simulink model "pendulumgui"  (R2016a)
settings: Solver=ode4  StartTime=0.0  StopTime=20  FixedStep=0.001  RelTol=1e-3
values from neighbouring files (symbols this model uses):
  c1 = str2double(sys_parameters{6})    [DIP_gui.m]    (also in paramters.m = 0.0001)
  c2 = str2double(sys_parameters{12})    [DIP_gui.m]    (also in paramters.m = 0.002)
  g = -9.8    [BP_linear.m]    (also in DIP_gui.m = str2double(sys_parameters{13}); paramters.m = 9.8)
  I1 = str2double(sys_parameters{5})    [DIP_gui.m]    (also in paramters.m = 0.0089)
  I2 = str2double(sys_parameters{11})    [DIP_gui.m]    (also in paramters.m = 0.0018)
  Jn1 = str2double(sys_parameters{4})    [DIP_gui.m]    (also in paramters.m = 2.8e-05)
  Jn2 = str2double(sys_parameters{10})    [DIP_gui.m]    (also in paramters.m = 2e-06)
  L = str2double(sys_parameters{14})    [DIP_gui.m]    (also in paramters.m = 0.38)
  l1 = str2double(sys_parameters{3})    [DIP_gui.m]    (also in paramters.m = 0.19)
  l2 = str2double(sys_parameters{9})    [DIP_gui.m]    (also in paramters.m = 0.115)
  m1 = str2double(sys_parameters{1})    [DIP_gui.m]    (also in paramters.m = 0.18)
  m2 = str2double(sys_parameters{7})    [DIP_gui.m]    (also in paramters.m = 0.1)
  n1 = str2double(sys_parameters{2})    [DIP_gui.m]    (also in paramters.m = 0.078)
  n2 = str2double(sys_parameters{8})    [DIP_gui.m]    (also in paramters.m = 0.05)
  T = 0.01    [paramters.m]
undefined symbols (not defined in the file or in its folder): a1, a2, m0
libraries: vrlib x6, simulink x1
settings Model: Creator=akhan  LastModifiedBy=akhan
settings SolverCC: SolverResetMethod=Robust
settings DataIOCC: LimitDataPoints=on  SaveFormat=Array
settings OptimizationCC: SimCompilerOptimization=on
settings DebuggingCC: SolverPrmCheckMsg=warning  MultiTaskRateTransMsg=warning
settings HardwareCC: ProdBitPerPointer=32  ProdLargestAtomicFloat=None  ProdIntDivRoundTo=Undefined  ProdEndianess=Unspecified  ProdWordSize=32  ProdHWDeviceType=32-bit Generic
settings ModelReferenceCC: PropagateSignalLabelsOutOfModel=off
settings ConfigComp: CovModelRefEnable=Off  CovSFcnEnable=off

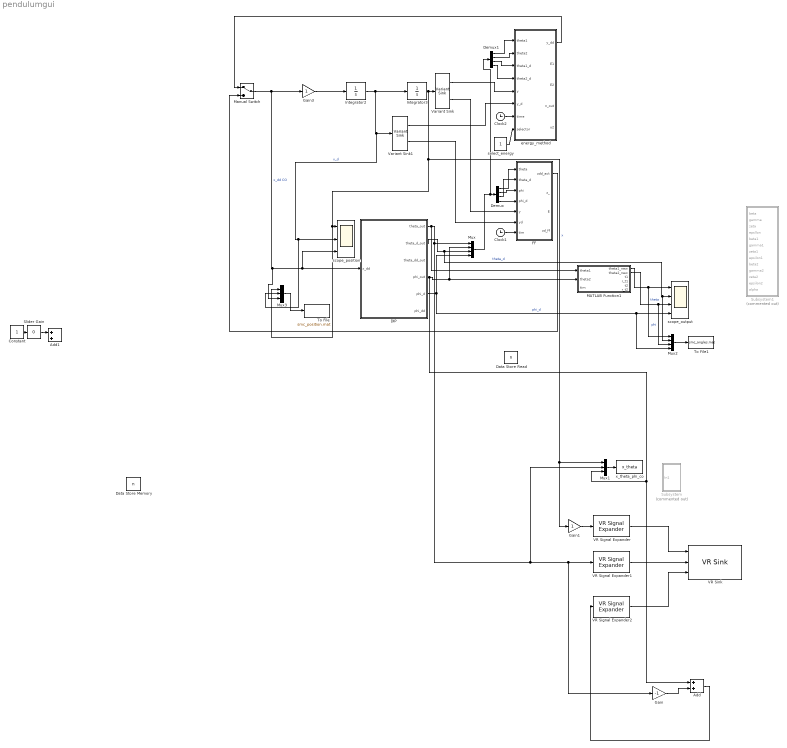
== system pendulumgui ==
  Add : Sum
  Add1 : Sum
  Clock1 : Clock
  Clock2 : Clock
  Constant : Constant
  DIP : Subsystem
  Data Store Memory : DataStoreMemory  DataStoreName=n  InitialValue=1  ShowAdditionalParam=off  OutDataTypeStr=double
  Data Store Read : DataStoreRead  DataStoreName=n  DataStoreElements=n
  Demux : Demux
  Demux1 : Demux
  FF : Subsystem
  Gain : Gain  Gain=-1
  Gain1 : Gain
  Gain3 : Gain
  Integrator2 : Integrator
  Integrator3 : Integrator  LimitOutput=on  UpperSaturationLimit=8  LowerSaturationLimit=-8
  MATLAB Function1 : MATLAB Function  TreatAsAtomicUnit=on
  Manual Switch : ManualSwitch
  Mux : Mux
  Mux1 : Mux  Inputs=3
  Mux2 : Mux
  Mux3 : Mux  Inputs=3
  Slider Gain : simulink/Math Operations/Slider Gain  low=-50  gain=0  high=50
  Subsystem : Subsystem  Commented=on
  Subsystem1 : Subsystem  Commented=on  mask{m0=0.8, m1=0.18, m2=0.10, l1=0.19, l2=0.115, a1=0.01, c1=0.2, a2=0.01, c2=0.2, g=9.8}
  To File : ToFile  Filename=smc_position.mat  SaveFormat=Timeseries
  To File1 : ToFile  Filename=smc_angles.mat  SaveFormat=Timeseries
  VR Signal Expander : vrlib/VR Signal Expander  outwidth=3  outidx=[1]
  VR Signal Expander1 : vrlib/VR Signal Expander  outwidth=4  outidx=[4]
  VR Signal Expander2 : vrlib/VR Signal Expander  outwidth=4  outidx=[4]
  VR Sink : vrlib/VR Sink  InstantiateOnLoad=on  SampleTime=0.05  ViewEnable=on  RemoteChange=off  RemoteView=off  FieldsWritten=slider_wpendulum.translation.3.1.1.double#first_arm.rotation.4.1.1.double#second_arm.rotation.4.1.1.double  WorldFileName=Double_Inverted_Pendullum_updated3.wrl  AutoView=off  VideoDimensions=[]  AllowVariableSize=off
  Variant Sink : VariantSink  ShowConditionOnBlock=on
  Variant Sink1 : VariantSink
  energy_method : MATLAB Function  TreatAsAtomicUnit=on
  scope_output : Scope  NumInputPorts=4
  scope_position : Scope  NumInputPorts=3
  select_energy : Constant
  x_theta_phi_co : ToWorkspace  VariableName=x_theta  SaveFormat=Timeseries  SampleTime=-1
  wires:
  Add/1 -> VR Signal Expander2/1
  Gain/1 -> Add/2
  DIP/4(phi_out) -> Mux1/3, Add/1, Mux/2, MATLAB Function1/2(theta2)
  Gain3/1 -> Integrator2/1
  DIP/5(phi_d) -> Mux/4, Mux2/4, scope_output/4  "phi_d"
  Constant/1 -> Slider Gain/1
  Slider Gain/1 -> Add1/1
  MATLAB Function1/2(theta2_new) -> Mux2/3, scope_output/3  "phi"
  select_energy/1 -> energy_method/8(selector)
  DIP/2(theta_d_out) -> Mux2/2, scope_output/2, Mux/3  "theta_d"
  Mux/1 -> Demux/1, Demux1/1
  Clock1/1 -> FF/7(tim)
  Clock2/1 -> energy_method/7(time)
  Demux1/1 -> energy_method/1(theta1)
  Demux1/2 -> energy_method/2(theta2)
  Demux1/3 -> energy_method/3(theta1_d)
  Demux1/4 -> energy_method/4(theta2_d)
  Variant Sink/1 -> energy_method/5(y)
  Variant Sink1/1 -> energy_method/6(y_d)
  Integrator2/1 -> Mux3/2, scope_position/2, Variant Sink1/1, Integrator3/1  "x_d"
  Manual Switch/1 -> Mux3/3, scope_position/3, DIP/1(x_dd), Gain3/1  "x_dd CO"
  energy_method/1(y_dd) -> Manual Switch/1
  DIP/1(theta_out) -> Mux/1, Mux1/2, Gain/1, VR Signal Expander1/1, MATLAB Function1/1(theta1)
  Integrator3/1 -> Mux3/1, scope_position/1, Mux1/1, Gain1/1, Variant Sink/1  "x"
  Variant Sink1/2 -> FF/6(yd)
  Demux/1 -> FF/1(theta)
  Demux/3 -> FF/2(theta_d)
  Demux/2 -> FF/3(phi)
  Demux/4 -> FF/4(phi_d)
  Variant Sink/2 -> FF/5(y)
  FF/1(zdd_act) -> Manual Switch/2
  Mux1/1 -> x_theta_phi_co/1
  VR Signal Expander/1 -> VR Sink/1
  VR Signal Expander1/1 -> VR Sink/2
  VR Signal Expander2/1 -> VR Sink/3
  Gain1/1 -> VR Signal Expander/1
  MATLAB Function1/1(theta1_new) -> Mux2/1, scope_output/1  "theta"
  Mux2/1 -> To File1/1
  Mux3/1 -> To File/1

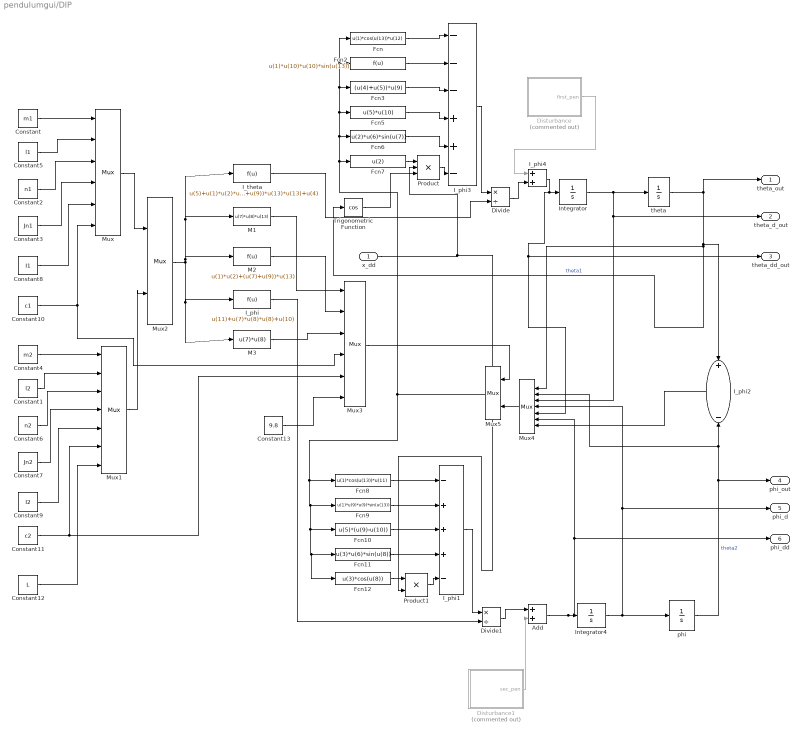
== system pendulumgui/DIP ==
  x_dd : Inport
  Add : Sum
  Constant : Constant  Value=m1
  Constant1 : Constant  Value=l2
  Constant10 : Constant  Value=c1
  Constant11 : Constant  Value=c2
  Constant12 : Constant  Value=L
  Constant13 : Constant  Value=9.8
  Constant2 : Constant  Value=n1
  Constant3 : Constant  Value=Jn1
  Constant4 : Constant  Value=m2
  Constant5 : Constant  Value=l1
  Constant6 : Constant  Value=n2
  Constant7 : Constant  Value=Jn2
  Constant8 : Constant  Value=I1
  Constant9 : Constant  Value=I2
  Disturbance : Subsystem  Commented=on
  Disturbance1 : Subsystem  Commented=on
  Divide : Product  Inputs=*/
  Divide1 : Product  Inputs=*/
  Fcn : Fcn  Expr=u(1)*cos(u(13))*u(12)
  Fcn10 : Fcn  Expr=u(5)*(u(9)-u(10))
  Fcn11 : Fcn  Expr=u(3)*u(6)*sin(u(8))
  Fcn12 : Fcn  Expr=u(3)*cos(u(8))
  Fcn2 : Fcn  Expr=u(1)*u(10)*u(10)*sin(u(13))
  Fcn3 : Fcn  Expr=(u(4)+u(5))*u(9)
  Fcn5 : Fcn  Expr=u(5)*u(10)
  Fcn6 : Fcn  Expr=u(2)*u(6)*sin(u(7))
  Fcn7 : Fcn  Expr=u(2)
  Fcn8 : Fcn  Expr=u(1)*cos(u(13))*u(11)
  Fcn9 : Fcn  Expr=u(1)*u(9)*u(9)*sin(u(13))
  I_phi : Fcn  Expr=u(11)+u(7)*u(8)*u(8)+u(10)
  I_phi1 : Sum  Inputs=-+++-
  I_phi2 : Sum  Inputs=+|-
  I_phi3 : Sum  Inputs=---++-
  I_phi4 : Sum
  I_theta : Fcn  Expr=u(5)+u(1)*u(2)*u(2)+(u(7)+u(9))*u(13)*u(13)+u(4)
  Integrator : Integrator
  Integrator4 : Integrator
  M1 : Fcn  Expr=u(7)*u(8)*u(13)
  M2 : Fcn  Expr=u(1)*u(2)+(u(7)+u(9))*u(13)
  M3 : Fcn  Expr=u(7)*u(8)
  Mux : Mux  Inputs=6
  Mux1 : Mux  Inputs=7
  Mux2 : Mux  Inputs=2
  Mux3 : Mux  Inputs=6
  Mux4 : Mux  Inputs=7
  Mux5 : Mux  Inputs=2
  Product : Product  Inputs=3
  Product1 : Product
  Trigonometric Function : Trigonometry  Operator=cos
  phi : Integrator  InitialCondition=-pi  WrapState=on
  theta : Integrator  InitialCondition=-pi+(pi/100)  WrapState=on
  theta_out : Outport
  theta_d_out : Outport  Port=2
  theta_dd_out : Outport  Port=3
  phi_out : Outport  Port=4
  phi_d : Outport  Port=5
  phi_dd : Outport  Port=6
  wires:
  Integrator4/1 -> Mux4/4, phi_d/1, phi/1
  Integrator/1 -> Mux4/3, theta_d_out/1, theta/1
  theta/1 -> Trigonometric Function/1, Mux4/1, I_phi2/1, theta_out/1  "theta1"
  phi/1 -> Mux4/2, I_phi2/2, phi_out/1  "theta2"
  Constant/1 -> Mux/1
  Constant5/1 -> Mux/2
  Constant2/1 -> Mux/3
  Constant3/1 -> Mux/4
  Constant8/1 -> Mux/5
  Constant10/1 -> Mux/6, Mux3/4
  Constant4/1 -> Mux1/1
  Constant1/1 -> Mux1/2
  Constant6/1 -> Mux1/3
  Constant7/1 -> Mux1/4
  Constant9/1 -> Mux1/5
  Constant11/1 -> Mux3/5, Mux1/6
  Mux/1 -> Mux2/1
  Mux1/1 -> Mux2/2
  Mux2/1 -> M3/1, I_phi/1, M2/1, I_theta/1, M1/1
  Constant12/1 -> Mux1/7
  M1/1 -> Mux3/1
  M2/1 -> Mux3/2
  M3/1 -> Mux3/3
  Constant13/1 -> Mux3/6
  I_phi3/1 -> Divide/1
  I_theta/1 -> Divide/2
  I_phi/1 -> Divide1/2
  Mux4/1 -> Mux5/2
  Mux3/1 -> Mux5/1
  I_phi1/1 -> Divide1/1
  Fcn/1 -> I_phi3/1
  Fcn2/1 -> I_phi3/2
  Fcn3/1 -> I_phi3/3
  Fcn5/1 -> I_phi3/4
  Fcn6/1 -> I_phi3/5
  Mux5/1 -> Fcn10/1, Fcn11/1, Fcn12/1, Fcn9/1, Fcn8/1, Fcn/1, Fcn2/1, Fcn3/1, Fcn5/1, Fcn6/1, Fcn7/1
  Fcn8/1 -> I_phi1/1
  Fcn9/1 -> I_phi1/2
  Fcn10/1 -> I_phi1/3
  Fcn11/1 -> I_phi1/4
  I_phi2/1 -> Mux4/7
  Product/1 -> I_phi3/6
  Fcn12/1 -> Product1/1
  Product1/1 -> I_phi1/5
  x_dd/1 -> Product1/2, Product/2
  Trigonometric Function/1 -> Product/3
  Fcn7/1 -> Product/1
  I_phi4/1 -> Mux4/5, theta_dd_out/1, Integrator/1
  Add/1 -> phi_dd/1, Mux4/6, Integrator4/1
  Divide1/1 -> Add/1
  Divide/1 -> I_phi4/2
  Disturbance/1(first_pen) -> I_phi4/1
  Disturbance1/1(sec_pen) -> Add/2

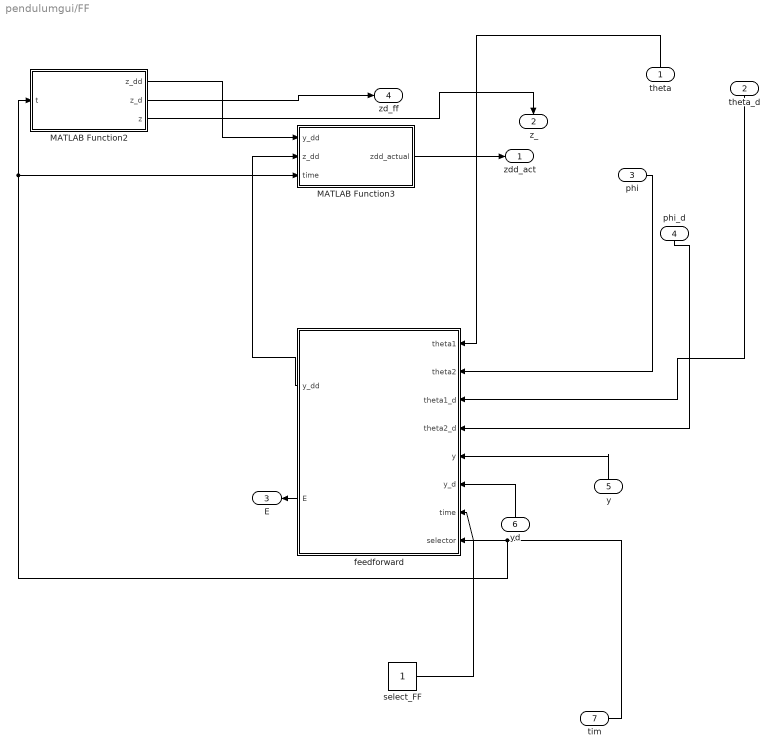
== system pendulumgui/FF ==
  theta : Inport
  theta_d : Inport  Port=2
  phi : Inport  Port=3
  phi_d : Inport  Port=4
  y : Inport  Port=5
  yd : Inport  Port=6
  tim : Inport  Port=7
  MATLAB Function2 : MATLAB Function  TreatAsAtomicUnit=on
  MATLAB Function3 : MATLAB Function  TreatAsAtomicUnit=on
  feedforward : MATLAB Function  TreatAsAtomicUnit=on
  select_FF : Constant
  zdd_act : Outport
  z_ : Outport  Port=2
  E : Outport  Port=3
  zd_ff : Outport  Port=4
  wires:
  feedforward/2(E) -> E/1
  y/1 -> feedforward/5(y)
  phi_d/1 -> feedforward/4(theta2_d)
  theta_d/1 -> feedforward/3(theta1_d)
  phi/1 -> feedforward/2(theta2)
  yd/1 -> feedforward/6(y_d)
  theta/1 -> feedforward/1(theta1)
  tim/1 -> MATLAB Function3/3(time), MATLAB Function2/1(t), feedforward/7(time)
  MATLAB Function3/1(zdd_actual) -> zdd_act/1
  MATLAB Function2/2(z_d) -> zd_ff/1
  MATLAB Function2/1(z_dd) -> MATLAB Function3/1(y_dd)
  MATLAB Function2/3(z) -> z_/1
  feedforward/1(y_dd) -> MATLAB Function3/2(z_dd)
  select_FF/1 -> feedforward/8(selector)

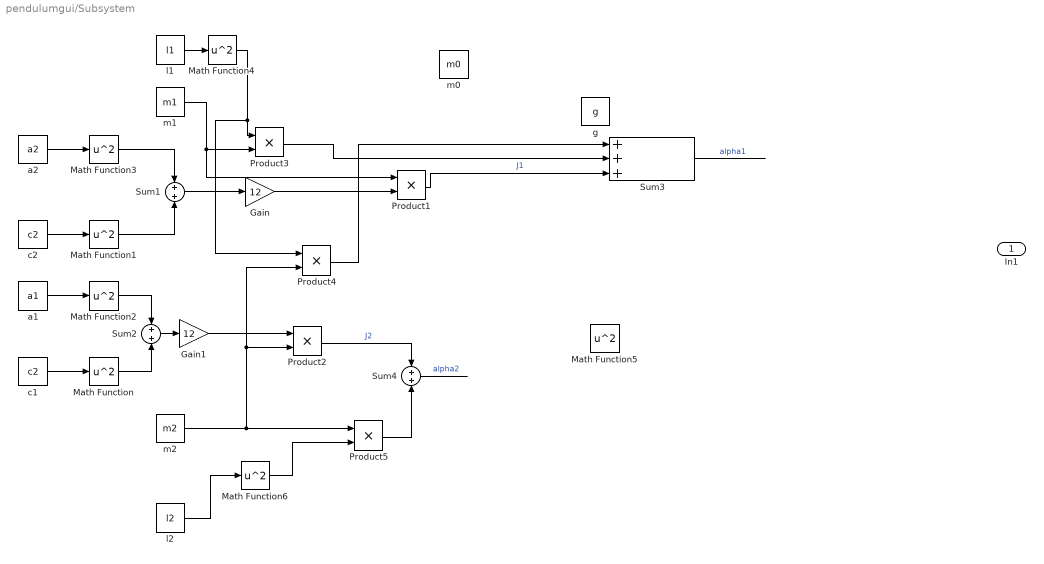
== system pendulumgui/Subsystem ==
  In1 : Inport
  Gain : Gain  Gain=12
  Gain1 : Gain  Gain=12
  Math Function{,1..6} (7 alike) : Math  Operator=square  SaturateOnIntegerOverflow=on
  Product{1..5} (5 alike) : Product
  Sum1 : Sum  Inputs=+|+
  Sum2 : Sum  Inputs=+|+
  Sum3 : Sum  Inputs=+++
  Sum4 : Sum  Inputs=+|+
  a1 : Constant  Value=a1
  a2 : Constant  Value=a2
  c1 : Constant  Value=c2
  c2 : Constant  Value=c2
  g : Constant  Value=g
  l1 : Constant  Value=l1
  l2 : Constant  Value=l2
  m0 : Constant  Value=m0
  m1 : Constant  Value=m1
  m2 : Constant  Value=m2
  wires:
  a2/1 -> Math Function3/1
  a1/1 -> Math Function2/1
  c2/1 -> Math Function1/1
  Math Function3/1 -> Sum1/1
  Math Function/1 -> Sum2/2
  Math Function1/1 -> Sum1/2
  Math Function2/1 -> Sum2/1
  m2/1 -> Product4/2, Product2/2, Product5/1
  m1/1 -> Product1/1, Product3/2
  c1/1 -> Math Function/1
  Product1/1 -> Sum3/3  "J1"
  Product3/1 -> Sum3/2
  l1/1 -> Math Function4/1
  Math Function4/1 -> Product4/1, Product3/1
  Product4/1 -> Sum3/1
  Sum3/1 -> ?  "alpha1"
  l2/1 -> Math Function6/1
  Sum1/1 -> Gain/1
  Gain/1 -> Product1/2
  Sum2/1 -> Gain1/1
  Gain1/1 -> Product2/1
  Math Function6/1 -> Product5/2
  Product2/1 -> Sum4/1  "J2"
  Product5/1 -> Sum4/2
  Sum4/1 -> ?  "alpha2"

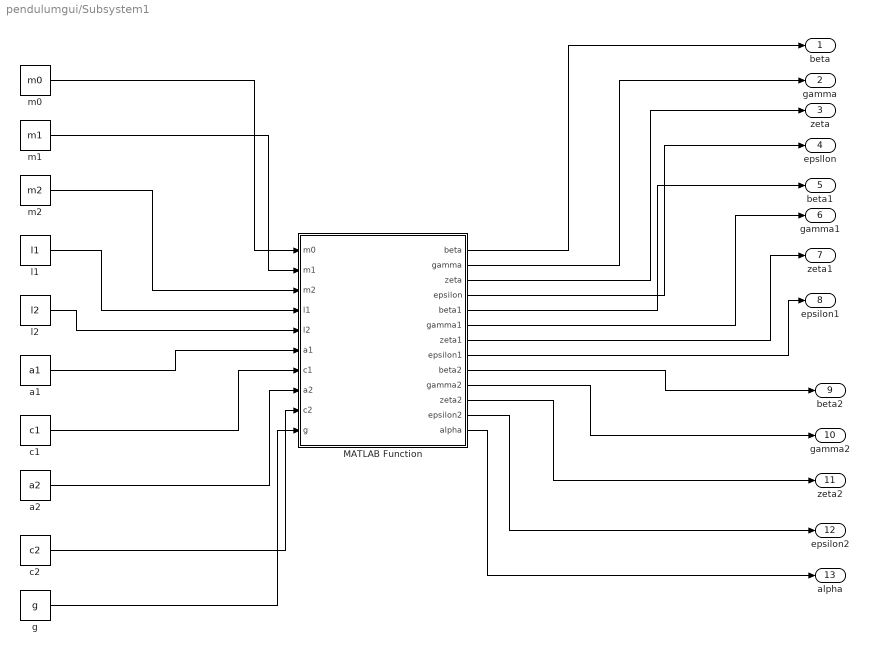
== system pendulumgui/Subsystem1 ==
  MATLAB Function : MATLAB Function  TreatAsAtomicUnit=on
  a1 : Constant  Value=a1
  a2 : Constant  Value=a2
  c1 : Constant  Value=c1
  c2 : Constant  Value=c2
  g : Constant  Value=g
  "l1 " : Constant  Value=l1
  l2 : Constant  Value=l2
  m0 : Constant  Value=m0
  m1 : Constant  Value=m1
  m2 : Constant  Value=m2
  beta : Outport
  gamma : Outport  Port=2
  zeta : Outport  Port=3
  epsllon : Outport  Port=4
  beta1 : Outport  Port=5
  gamma1 : Outport  Port=6
  zeta1 : Outport  Port=7
  epsilon1 : Outport  Port=8
  beta2 : Outport  Port=9
  gamma2 : Outport  Port=10
  zeta2 : Outport  Port=11
  epsilon2 : Outport  Port=12
  alpha : Outport  Port=13
  wires:
  m1/1 -> MATLAB Function/2(m1)
  m0/1 -> MATLAB Function/1(m0)
  "l1 "/1 -> MATLAB Function/4(l1)
  c2/1 -> MATLAB Function/9(c2)
  MATLAB Function/1(beta) -> beta/1
  MATLAB Function/10(gamma2) -> gamma2/1
  MATLAB Function/11(zeta2) -> zeta2/1
  MATLAB Function/5(beta1) -> beta1/1
  MATLAB Function/12(epsilon2) -> epsilon2/1
  MATLAB Function/9(beta2) -> beta2/1
  MATLAB Function/2(gamma) -> gamma/1
  MATLAB Function/7(zeta1) -> zeta1/1
  MATLAB Function/6(gamma1) -> gamma1/1
  MATLAB Function/3(zeta) -> zeta/1
  MATLAB Function/4(epsilon) -> epsllon/1
  MATLAB Function/8(epsilon1) -> epsilon1/1
  m2/1 -> MATLAB Function/3(m2)
  l2/1 -> MATLAB Function/5(l2)
  a1/1 -> MATLAB Function/6(a1)
  c1/1 -> MATLAB Function/7(c1)
  a2/1 -> MATLAB Function/8(a2)
  g/1 -> MATLAB Function/10(g)
  MATLAB Function/13(alpha) -> alpha/1

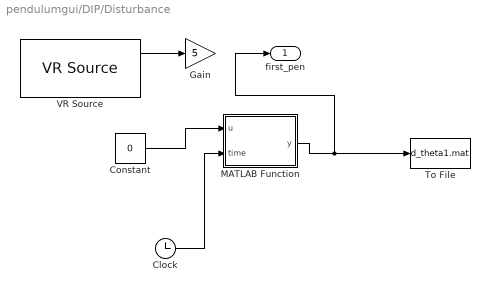
== system pendulumgui/DIP/Disturbance ==
  Clock : Clock
  Constant : Constant  Value=0
  Gain : Gain  Gain=5
  MATLAB Function : MATLAB Function  TreatAsAtomicUnit=on
  To File : ToFile  Filename=d_theta1.mat  SaveFormat=Timeseries
  VR Source : vrlib/VR Source  InstantiateOnLoad=on  SampleTime=T  ViewEnable=on  RemoteChange=off  RemoteView=off  FieldsRead=first_arm_touch.isActive#second_arm_touch.isActive  WorldFileName=Double_Inverted_Pendullum_updated3.wrl  AutoView=off  VideoDimensions=[]  AllowVariableSize=off
  first_pen : Outport
  wires:
  VR Source/1 -> Gain/1
  MATLAB Function/1(y) -> first_pen/1, To File/1
  Constant/1 -> MATLAB Function/1(u)
  Clock/1 -> MATLAB Function/2(time)

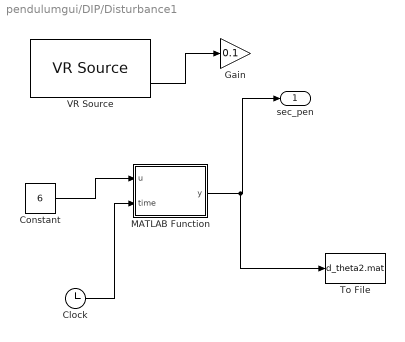
== system pendulumgui/DIP/Disturbance1 ==
  Clock : Clock
  Constant : Constant  Value=6
  Gain : Gain  Gain=0.1  OutDataTypeStr=double
  MATLAB Function : MATLAB Function  TreatAsAtomicUnit=on
  To File : ToFile  Filename=d_theta2.mat  SaveFormat=Timeseries
  VR Source : vrlib/VR Source  InstantiateOnLoad=on  SampleTime=T  ViewEnable=on  RemoteChange=off  RemoteView=off  FieldsRead=first_arm_touch.isActive.1.1.1.logical#second_arm_touch.isActive.1.1.1.logical  WorldFileName=Double_Inverted_Pendullum_updated3.wrl  AutoView=off  VideoDimensions=[]  AllowVariableSize=off
  sec_pen : Outport
  wires:
  VR Source/2 -> Gain/1
  Constant/1 -> MATLAB Function/1(u)
  Clock/1 -> MATLAB Function/2(time)
  MATLAB Function/1(y) -> To File/1, sec_pen/1

== matlab function pendulumgui/DIP/Disturbance/MATLAB Function ==
  data: u input; y output; time input
function y = fcn(u,time)
%#codegen
if time>5&&time<6
y = u;
else
    y=0;
end

== matlab function pendulumgui/Subsystem1/MATLAB Function ==
  data: m0 input; beta output; m1 input; m2 input; l1 input; l2 input; a1 input; c1 input; a2 input; c2 input; g input; gamma output; zeta output; epsilon output; beta1 output; gamma1 output; zeta1 output; epsilon1 output; beta2 output; gamma2 output; zeta2 output; epsilon2 output; alpha output
function [beta,gamma,zeta,epsilon,beta1,gamma1,zeta1,epsilon1,beta2,gamma2,zeta2,epsilon2,alpha] = fcn(m0,m1,m2,l1,l2,a1,c1,a2,c2,g)
%#codegen
J1=m1*((a1*a1)+(c1*c1))/12;
J2=m2*((a2*a2)+(c2*c2))/12;
J1=0.0089;
J2=0.0018;
alpha1 = (m1*l1*l1)+(m2*l1*l1)+J1;
alpha2 = (m2*l2*l2)+J2;

beta1 = (m1*l1)+(m2*l1);
beta2 = m2*l2;

gamma1 = m2*l1*l2;
gamma2 = gamma1;

zeta1 = gamma1;
zeta2 = gamma1;

epsilon1 = ((m1*l1)+(m2*l1))*g;
epsilon2 = beta2;

alpha = m0+m1+m2;
beta = beta1;
gamma = epsilon2;
zeta = beta;
epsilon = gamma;

beta1 = beta1/alpha1;
gamma1 = gamma1/alpha1;
zeta1 = zeta1/alpha1;
epsilon1 = epsilon1/alpha1;

beta2 = beta2/alpha2;
gamma2 = gamma2/alpha2;
zeta2 = zeta2/alpha2;
epsilon2 = epsilon2/alpha2;

beta = beta/alpha;
gamma = gamma/alpha;
zeta = zeta/alpha;
epsilon = epsilon/alpha;

== matlab function pendulumgui/MATLAB Function1 ==
  data: theta1 input; theta1_new output; theta2 input; theta2_new output; t1 output; r_t1 output; t2 output; r_t2 output; tim input
function [theta1_new,theta2_new,t1,r_t1,t2,r_t2] = fcn(theta1,theta2,tim)
%#codegen

theta1_new = cos(theta1);
theta1_new = acosd(theta1_new);
theta2_new = cos(theta2);
theta2_new = acosd(theta2_new);


% if theta1>2*pi||theta1<(-2*pi)
%     t1 = mod(theta1,2*pi);
%     r_t1 = 1;
% else r_t1 =0;
%     t1 = theta1;
% end
% 
% if theta2>2*pi||theta2<(-2*pi)
%     t2 = mod(theta2,2*pi);
%     r_t2 = 1;
% else r_t2 =0;
%     t2 = theta2;
% end

if tim==0
    r_t1 = 1;
    r_t2 = 1;
   t1 = 0;
   t2 = 0;
else
    r_t1=0;
    r_t2=0;
    t1=0;
    t2=0;
end

== matlab function pendulumgui/DIP/Disturbance1/MATLAB Function ==
  data: u input; y output; time input
function y = fcn(u,time)
%#codegen
if time>5&&time<7
y = u;
else
    y=0;
end

== matlab function pendulumgui/FF/feedforward ==
  data: theta1 input; theta2 input; theta1_d input; theta2_d input; y input; y_d input; y_dd output; time input; E output; selector input
function [y_dd,E] =fcn(theta1,theta2,theta1_d,theta2_d,y,y_d,time,selector)
%#codegen

m1 = 0.18;
n1 = 0.078;
l1 = 0.19;
Jn1 = 2.8e-5;
I1 = 0.0089;
c1 = 0.0001;
m2 = 0.1;
n2 = 0.05;
l2 = 0.115;
Jn2 = 2e-6;
I2 = 0.0018;
c2 = 0.002;
g = 9.8;
L = 0.38;
alpha_theta = 1;
alpha_phi = 2;
alpha_theta_d = 1.2;
alpha_phi_d = 20;

E = alpha_theta*abs(theta1)+alpha_phi*abs(theta2);
E = alpha_theta_d*abs(theta1_d)+alpha_phi_d*abs(theta2_d);
E1 = 1/2*I1*theta1_d^2;
E1 = E1 + m1*g*l1*(cos(theta1)-1);

E2 = 1/2*I2*theta2_d^2;
E2 = E2 + m2*g*l2*(cos(theta2)-1);

I_theta = I1 +m1*(l1^2)+m2*(L^2)+n2*(L^2)+Jn1;
M1 = m2*l2*L;
M2 = m1*l1+m2*L+n2*L;
I_phi = I2+m2*(l2*l2)+Jn2;
M3=m2*l2;

%Calculating energy

t_exit=15;
ua1 = 14;
%X_dd in first phase



if time>1.6
    n_out = 3;
x3 = [theta1;theta1_d;theta2;theta2_d;y;y_d];

a21 = -M2*I_phi*g;
a_den =(I_phi*I_theta-(M1^2));
a21 = a21/a_den;

a22 = -(M1*c2+I_phi*(c1+c2));
a22 = a22/a_den;

a23 = M1*M3*g/a_den;

a24 = I_phi*c1 + M1*c2;
a24 = a24/a_den;

a41 = M1*M2*g/a_den;

a42 = I_theta*c2 + M1*(c1+c2);
a42 = a42/a_den;


a43 = -(M3*I_theta)*g/a_den;

a44 = -(I_theta*c2+M1*c1);
a44 = a44/a_den;

b2 = M1*M3-M2*I_phi;
b2 = b2/a_den;

b4 = M1*M2-M3*I_theta;
b4 = b4/a_den;

A3 = [0 1 0 0 0 0
     a21 a22 a23 a24 0 0
     0 0 0 1 0 0
     a41 a42 a43 a44 0 0
     0 0 0 0 0 1
     0 0 0 0 0 0];
 B3 = [0;b2;0;b4;0;1];
    A3 =[         0    1.0000         0         0         0         0
   28.8552   -0.1581   -5.0889    0.1549         0         0
         0         0         0    1.0000         0         0
  -40.3575    0.8612   43.1873   -0.8567         0         0
         0         0         0         0         0         1
         0         0         0         0         0         0];
 
 ep3 = 1;
 K3 = 10;
 R3=3;
 
% P3 = care(A3+ep3*eye(6),B3,eye(6));


P3 = 1.0e+03 *[3.3164    0.0753   -5.1074   -0.7356   -0.1996   -0.2951
                0.0753    0.0099   -0.0443   -0.0057    0.0097    0.0097
               -5.1074   -0.0443    8.5062    1.2307    0.4325    0.5997
               -0.7356   -0.0057    1.2307    0.1782    0.0634    0.0877
               -0.1996    0.0097    0.4325    0.0634    0.0506    0.0518
               -0.2951    0.0097    0.5997    0.0877    0.0518    0.0641];


S3 = (B3')*P3;


sigma_3 = S3*x3;

u3_1 = -inv(S3*B3);
u3_2 = S3*A3*x3;
u3_3 = R3*sign(sigma_3);
u3_4 = K3*sigma_3;
u3 = u3_1*(u3_2+u3_3+u3_4);
% gain = -[ -81.4700   -7.0211   76.8723   10.3521    0.1513    0.4473];
gain = -[ -360.2187  -19.7350  431.6744   65.4821    3.1623    7.3102];
%0 IS SMC and anything else is LQR
if selector==0
    y_dd = u3;
else
    y_dd = gain*x3; 
end

u2 = 0;
else
    y_dd = 0;
    n_out = 3;
    u2= 0;
    
end

== matlab function pendulumgui/FF/MATLAB Function2 ==
  data: t input; z_dd output; z_d output; z output
function [z_dd,z_d,z]  = fcn(t)
%#codegen



% p =[   -0.2007
%     0.1709
%     0.3038
%     0.1094];
% T = 1.8;


p=[  0.0859
    0.1996
   -0.0939
   -0.1516];
T=2.2;
if t==2.5
    j=5;
end
a0 = -p(1)-p(3);
a1 = -p(2)-p(4);

z = a0+a1*cos(pi*t/T);
z_d = (-a1*pi/T)*sin(pi*t/T);
z_dd = (-a1*pi*pi/T^2)*cos(pi*t/T);

for i=2:5
    z = z + p(i-1)*cos(i*pi*t/T);
    z_d = z_d -(p(i-1)*i*pi/T)*sin(i*pi*t/T);
    z_dd = z_dd-(p(i-1)*i*i*pi*pi/T^2)*cos(i*pi*t/T);
end

end

== matlab function pendulumgui/FF/MATLAB Function3 ==
  data: y_dd input; zdd_actual output; z_dd input; time input
function zdd_actual  = fcn(y_dd,z_dd,time)
%#codegen
if time>1.6
    zdd_actual = z_dd;
else
    zdd_actual = y_dd;
end

== matlab function pendulumgui/energy_method ==
  data: theta1 input; theta2 input; theta1_d input; theta2_d input; y input; y_d input; y_dd output; E1 output; E2 output; time input; n data_store_memory; n_out output; u2 output; selector input
function [y_dd,E1,E2,n_out,u2]=fcn(theta1,theta2,theta1_d,theta2_d,y,y_d,time,selector)
%#codegen
global n;
m1 = 0.18;
n1 = 0.078;
l1 = 0.19;
Jn1 = 2.8e-5;
I1 = 0.0089;
c1 = 0.0001;




m2 = 0.1;
n2 = 0.05;
l2 = 0.115;
Jn2 = 2e-6;
I2 = 0.0018;
c2 = 0.002;

g = 9.8;
L = 0.38;

E1 = 1/2*I1*theta1_d^2;
E1 = E1 + m1*g*l1*(cos(theta1)-1);

E2 = 1/2*I2*theta2_d^2;
E2 = E2 + m2*g*l2*(cos(theta2)-1);

I_theta = I1 +m1*(l1^2)+m2*(L^2)+n2*(L^2)+Jn1;
M1 = m2*l2*L;
M2 = m1*l1+m2*L+n2*L;
I_phi = I2+m2*(l2*l2)+Jn2;
M3=m2*l2;

%Calculating energy

t_exit=15;
ua1 = 14;
%X_dd in first phase
% if cos(theta1)<0.94


if n==1

    u_theta = ua1*sign(E1*theta1_d*cos(theta1));
    y_dd = u_theta;
u2 = 0;

 
if time==0.8
n=2;
end
n_out = 1;
elseif n==2
    n_out = 2;
%X_dd in second phase

A2 = [0 1 0 0
     M2*g/I_theta -((c1+c2)/I_theta) 0 0
     0 0 0 1
     0 0 0 0];
 B2 = [0;-M2/I_theta;0;1];
 ep2 = 1;

P =[229.7444   45.7155   56.6863   60.8077
   45.7155    9.2259   11.4113   12.2074
   56.6863   11.4113   27.8115   20.5373
   60.8077   12.2074   20.5373   20.8653];



S2 = (B2')*P;


x2 = [theta1;theta1_d;y;y_d];

sigma_2 = S2*x2;
R2 = 3;
K2 = 1;
u1_1 = -1/(S2*B2);
u1_2 = S2*A2*x2;
u1_3 = R2*sign(sigma_2);
u1_4 = K2*sigma_2;
u1 = u1_1*(u1_2+u1_3+u1_4);
u1 =  -[-27.5833   -5.6714   -1.0000   -2.1516];
u1 = u1*x2;

%energy bsed for pen2
A11 = I_theta;
A22 = I_phi;
A12 = M1*cos(theta1-theta2);
A21 = A12;


f11 =M1*(theta2_d^2)*sin(theta1-theta2)+(c1+c2)*theta1_d;
f11 = f11-c2*theta2_d-M2*g*sin(theta1);
f12 = M2*cos(theta1);
f21 = -M1*(theta1_d^2)*sin(theta1-theta2);
f21 = f21-c2*(theta1_d-theta2_d)-M3*g*sin(theta2);
f22 = M3*cos(theta2);


E2 = 1/2*I2*theta2_d^2;
E2 = E2 + m2*g*l2*(cos(theta2)-1);
mu = pi/12;
ua2 = 50;
cond11 = (sin(theta2)*theta2_d)<0;
cond12 = cos(theta2)<cos(mu);

cond21 = (sin(theta2)*theta2_d)>=0;
cond22  = cond12;
cond3 = cos(theta2)>=cos(mu);
if cond11&&cond12
    uz2 = ua2*sign(E2*theta2_d*cos(theta2));
elseif cond21&&cond22
    uz2 = 0;
elseif cond3
    uz2 = 0;
else uz2 = 0;
end
u2_num_1 = (uz2+L*(theta1_d^2)*sin(theta1));
u2_num_1 = u2_num_1*(A11*A22-A12*A21);
u2_num_2 = (A12*f21-A22*f11)*L*cos(theta1);
u2_num = u2_num_1 -u2_num_2;
u2_den = (A12*f22-A22*f12)*L*cos(theta1);
u2_den = u2_den+ A11*A22 - A12*A21;
u2 = u2_num/u2_den;

if abs(u2)>3
    u2 =3*sign(u2);
end
    
y_dd = (0.85*u1)+u2;
if cos(theta2)>0.90&&abs(theta2_d)<1.5
% if time==2.89
    n = 3;
    y_dd = u1;
end
%Step 3 Controller
elseif n==3
    n_out = 3;
x3 = [theta1;theta1_d;theta2;theta2_d;y;y_d];

a21 = -M2*I_phi*g;
a_den =(I_phi*I_theta-(M1^2));
a21 = a21/a_den;

a22 = -(M1*c2+I_phi*(c1+c2));
a22 = a22/a_den;

a23 = M1*M3*g/a_den;

a24 = I_phi*c1 + M1*c2;
a24 = a24/a_den;

a41 = M1*M2*g/a_den;

a42 = I_theta*c2 + M1*(c1+c2);
a42 = a42/a_den;


a43 = -(M3*I_theta)*g/a_den;

a44 = -(I_theta*c2+M1*c1);
a44 = a44/a_den;

b2 = M1*M3-M2*I_phi;
b2 = b2/a_den;

b4 = M1*M2-M3*I_theta;
b4 = b4/a_den;

A3 = [0 1 0 0 0 0
     a21 a22 a23 a24 0 0
     0 0 0 1 0 0
     a41 a42 a43 a44 0 0
     0 0 0 0 0 1
     0 0 0 0 0 0];
 B3 = [0;b2;0;b4;0;1];
 A3 =   [0    1.0000         0         0         0         0
   28.8552   -0.1581   -5.0889    0.1549         0         0
         0         0         0    1.0000         0         0
  -40.3575    0.8612   43.1873   -0.8567         0         0
         0         0         0         0         0    1.0000
         0         0         0         0         0         0];
 
 ep3 = 1;
 K3 = 10;
 R3=3;
 
% P3 = care(A3+ep3*eye(6),B3,eye(6));


P3 = 1.0e+03 *[3.3164    0.0753   -5.1074   -0.7356   -0.1996   -0.2951
                0.0753    0.0099   -0.0443   -0.0057    0.0097    0.0097
               -5.1074   -0.0443    8.5062    1.2307    0.4325    0.5997
               -0.7356   -0.0057    1.2307    0.1782    0.0634    0.0877
               -0.1996    0.0097    0.4325    0.0634    0.0506    0.0518
               -0.2951    0.0097    0.5997    0.0877    0.0518    0.0641];


S3 = (B3')*P3;


sigma_3 = S3*x3;

u3_1 = -inv(S3*B3);
u3_2 = S3*A3*x3;
u3_3 = R3*sign(sigma_3);
u3_4 = K3*sigma_3;
u3 = u3_1*(u3_2+u3_3+u3_4);
% gain = -[-81.4700   -7.0211   76.8723   10.3521    0.1513    0.4473];
gain = -[ -360.2187  -19.7350  431.6744   65.4821    3.1623    7.3102];


%0 IS SMC and anything else is LQR
if selector==0
    y_dd = u3;
else
    y_dd = gain*x3; 
end

u2 = 0;
else
    y_dd = 50;
    n_out = 3;
    u2= 0;
    
end
